simulink model "rocket"  (R2023a)
settings: Solver=FixedStepAuto  StartTime=0.0  StopTime=80  FixedStep=1/24  MaxStep=1.2  RelTol=1e-3
values from neighbouring files (symbols this model uses):
  arm_finne = 55    [rocket_variables.m]
  dry_mass = 25000    [rocket_variables.m]
  F_max = 845000    [rocket_variables.m]
  fuel_mass = 0    [rocket_variables.m]
  gravitational_constant = 6.6743E-11    (= 6.6743e-11)    [rocket_variables.m]
  h0 = 10000    [rocket_variables.m]
  h_ref = -1    [rocket_variables.m]
  J = dry_mass*L*L / 12    (= 10208333.3333)    [rocket_variables.m]
  k = 5.47    [rocket_variables.m]
  Kd1 = Kd    [rocket_variables.m]
  Kd_theta = 550000    [rocket_variables.m]
  Ki1 = Ki    [rocket_variables.m]
  Ki_theta = 125000    [rocket_variables.m]
  Kp1 = Kp    [rocket_variables.m]
  Kp_theta = 500000    [rocket_variables.m]
  mass_earth = 5.972E24    (= 5.972e+24)    [rocket_variables.m]
  mass_flow_engine = 1451.5    [rocket_variables.m]
  radius_earth = 6371000    [rocket_variables.m]
  theta_0 = pi/12    (= 0.261799387799)    [rocket_variables.m]
  theta_dot_0 = 0    [rocket_variables.m]
  theta_ref = 0    [rocket_variables.m]
  v_0 = -211    [rocket_variables.m]
libraries: embmathops x2
settings Model: Creator=eriknymobohne  LastModifiedBy=eriknymobohne

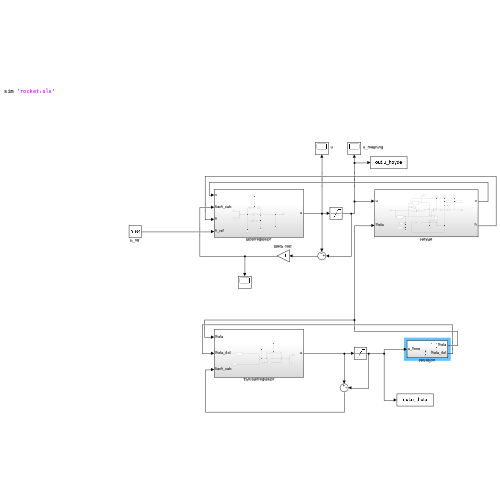
[thumbnail: Simulink's stored preview of the top-level diagram]
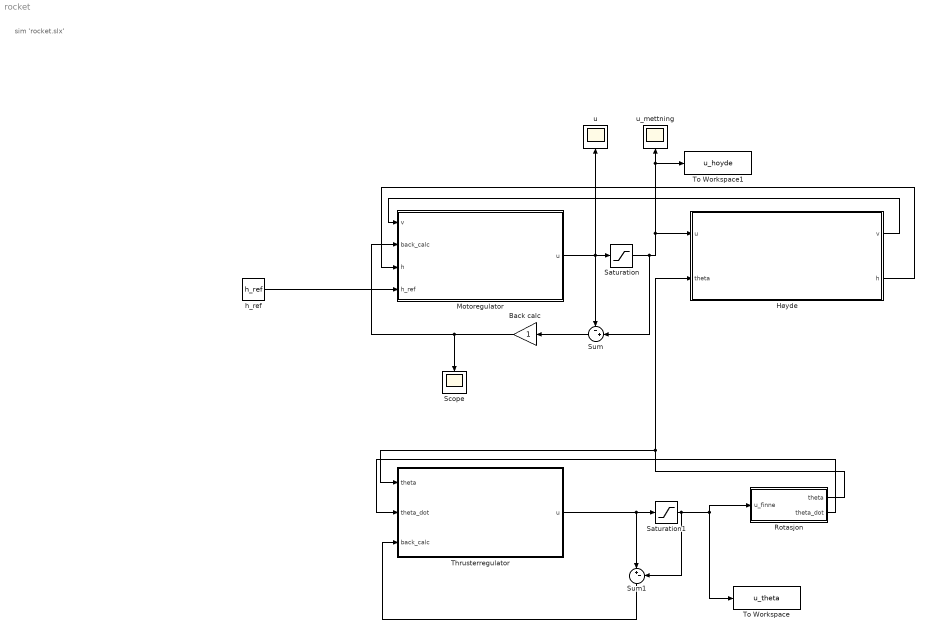
== system rocket ==
  note: sim 'rocket.slx'
  Back calc : Gain
  Høyde : Subsystem
  Motoregulator : Subsystem
  Rotasjon : Subsystem
  Saturation : Saturate  UpperLimit=F_max  LowerLimit=0
  Saturation1 : Saturate  UpperLimit=10000  LowerLimit=-10000
  Scope : Scope
  Sum : Sum  Inputs=-+|
  Sum1 : Sum  Inputs=|+-
  Thrusterregulator : Subsystem
  To Workspace : ToWorkspace  VariableName=u_theta  SaveFormat=Timeseries  SampleTime=-1
  To Workspace1 : ToWorkspace  VariableName=u_hoyde  SaveFormat=Timeseries  SampleTime=-1
  h_ref : Constant  Value=h_ref
  u : Scope
  u_mettning : Scope
  wires:
  Motoregulator/1(u) -> Saturation/1, Sum/1, u/1
  Saturation/1 -> To Workspace1/1, u_mettning/1, Høyde/1(u), Sum/2
  Sum/1 -> Back calc/1
  Back calc/1 -> Motoregulator/2(back_calc), Scope/1
  Høyde/2(h) -> Motoregulator/3(h)
  h_ref/1 -> Motoregulator/4(h_ref)
  Høyde/1(v) -> Motoregulator/1(v)
  Thrusterregulator/1(u) -> Sum1/1, Saturation1/1
  Sum1/1 -> Thrusterregulator/3(back_calc)
  Rotasjon/1(theta) -> Høyde/2(theta), Thrusterregulator/1(theta)
  Rotasjon/2(theta_dot) -> Thrusterregulator/2(theta_dot)
  Saturation1/1 -> Sum1/2, To Workspace/1, Rotasjon/1(u_finne)

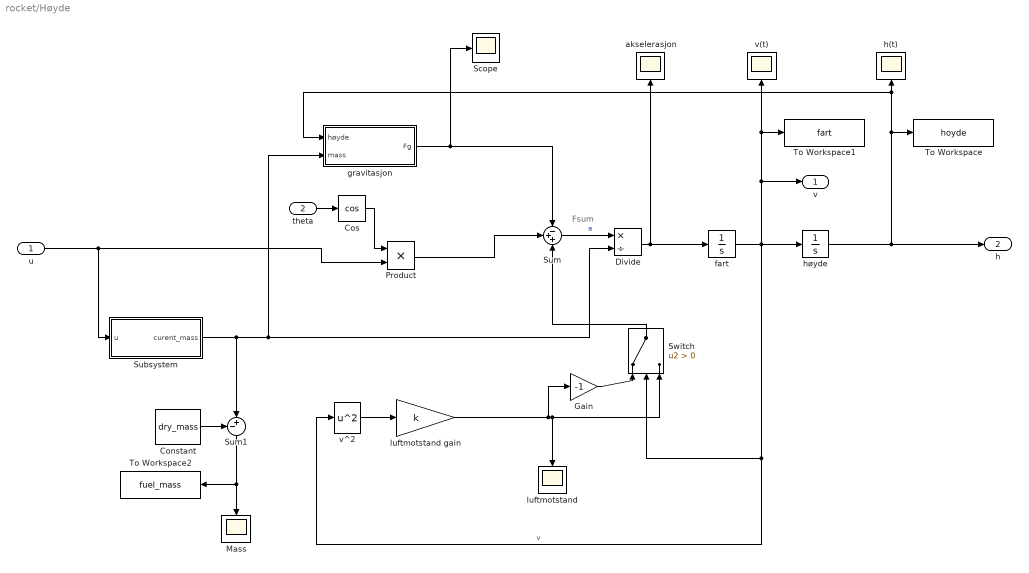
== system rocket/Høyde ==
  note: Fsum
  u : Inport
  theta : Inport  Port=2
  Constant : Constant  Value=dry_mass
  Cos : Trigonometry  Operator=cos
  Divide : Product  Inputs=*/
  Gain : Gain  Gain=-1
  Mass : Scope
  Product : Product
  Scope : Scope
  Subsystem : Subsystem
  Sum : Sum  Inputs=-++
  Sum1 : Sum  Inputs=-+|
  Switch : Switch  Criteria=u2 > Threshold  SaturateOnIntegerOverflow=off  InputSameDT=off
  To Workspace : ToWorkspace  VariableName=hoyde  SaveFormat=Timeseries  SampleTime=-1
  To Workspace1 : ToWorkspace  VariableName=fart  SaveFormat=Timeseries  SampleTime=-1
  To Workspace2 : ToWorkspace  VariableName=fuel_mass  SaveFormat=Timeseries  SampleTime=-1
  akselerasjon : Scope
  fart : Integrator  InitialCondition=v_0
  gravitasjon : Subsystem
  h(t) : Scope
  høyde : Integrator  InitialCondition=h0
  luftmotstand : Scope
  luftmotstand gain : Gain  Gain=k
  v(t) : Scope
  v^2 : Math  Operator=square
  v : Outport
  h : Outport  Port=2
  wires:
  fart/1 -> Switch/2, v^2/1, v/1, v(t)/1, To Workspace1/1, høyde/1  "v"
  v^2/1 -> luftmotstand gain/1
  luftmotstand gain/1 -> Switch/3, luftmotstand/1, Gain/1
  høyde/1 -> h/1, gravitasjon/1(høyde), h(t)/1, To Workspace/1
  Product/1 -> Sum/2
  theta/1 -> Cos/1
  u/1 -> Subsystem/1(u), Product/2
  Cos/1 -> Product/1
  gravitasjon/1(Fg) -> Scope/1, Sum/1
  Sum/1 -> Divide/1  "a"
  Subsystem/1(curent_mass) -> Sum1/2, Divide/2, gravitasjon/2(mass)
  Divide/1 -> fart/1, akselerasjon/1
  Switch/1 -> Sum/3
  Gain/1 -> Switch/1
  Constant/1 -> Sum1/1
  Sum1/1 -> To Workspace2/1, Mass/1

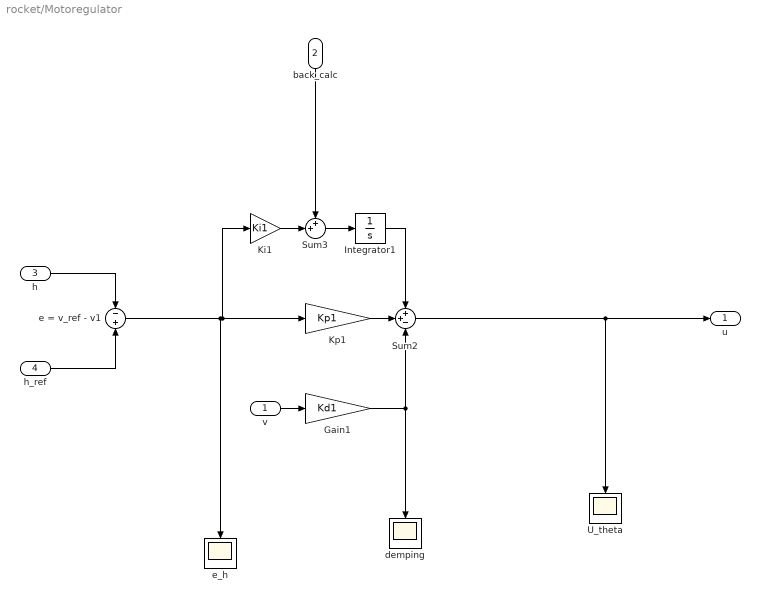
== system rocket/Motoregulator ==
  v : Inport
  back_calc : Inport  Port=2
  h : Inport  Port=3
  h_ref : Inport  Port=4
  Gain1 : Gain  Gain=Kd1
  Integrator1 : Integrator
  Ki1 : Gain  Gain=Ki1
  Kp1 : Gain  Gain=Kp1
  Sum2 : Sum  Inputs=++-
  Sum3 : Sum  Inputs=++|
  U_theta : Scope
  demping : Scope
  e = v_ref - v1 : Sum  Inputs=-|+
  e_h : Scope
  u : Outport
  wires:
  Integrator1/1 -> Sum2/1
  e = v_ref - v1/1 -> Ki1/1, Kp1/1, e_h/1
  Sum3/1 -> Integrator1/1
  h/1 -> e = v_ref - v1/1
  Kp1/1 -> Sum2/2
  Ki1/1 -> Sum3/2
  h_ref/1 -> e = v_ref - v1/2
  Sum2/1 -> U_theta/1, u/1
  back_calc/1 -> Sum3/1
  v/1 -> Gain1/1
  Gain1/1 -> Sum2/3, demping/1

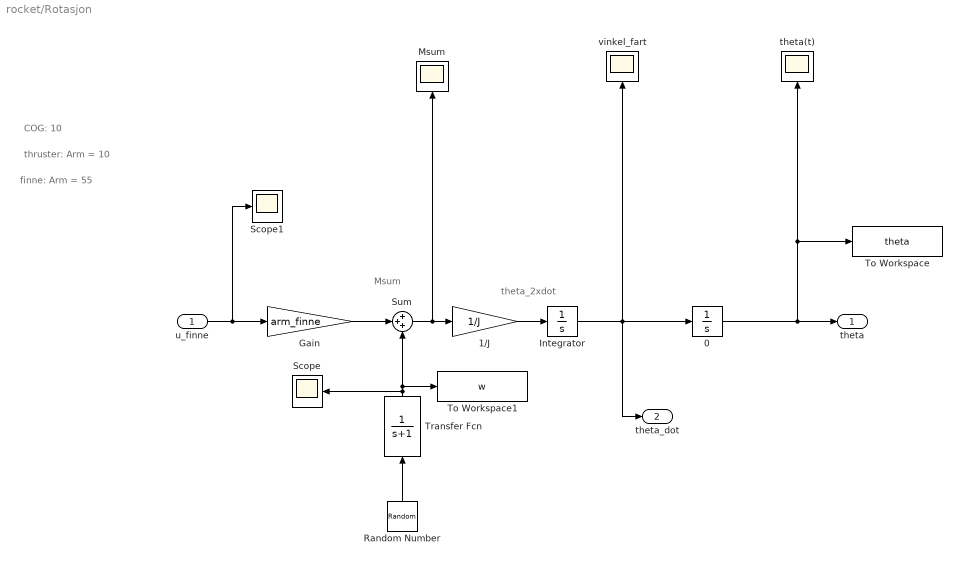
== system rocket/Rotasjon ==
  note: finne: Arm = 55
  note: COG: 10
  note: thruster: Arm = 10
  note: theta_2xdot
  note: Msum
  u_finne : Inport
  0 : Integrator  InitialCondition=theta_0
  1/J : Gain  Gain=1/J
  Gain : Gain  Gain=arm_finne
  Integrator : Integrator  InitialCondition=theta_dot_0
  Msum : Scope
  Random Number : RandomNumber  Mean=1000/2  Variance=10000000000  Seed=100000  SampleTime=1/24
  Scope : Scope
  Scope1 : Scope
  Sum : Sum  Inputs=+++
  To Workspace : ToWorkspace  VariableName=theta  SaveFormat=Timeseries  SampleTime=-1
  To Workspace1 : ToWorkspace  VariableName=w  SaveFormat=Timeseries  SampleTime=-1
  Transfer Fcn : TransferFcn  Denominator=[1 1]
  theta(t) : Scope
  vinkel_fart : Scope
  theta : Outport
  theta_dot : Outport  Port=2
  wires:
  0/1 -> theta(t)/1, To Workspace/1, theta/1
  Integrator/1 -> 0/1, vinkel_fart/1, theta_dot/1
  Sum/1 -> Msum/1, 1/J/1
  1/J/1 -> Integrator/1
  u_finne/1 -> Scope1/1, Gain/1
  Gain/1 -> Sum/2
  Random Number/1 -> Transfer Fcn/1
  Transfer Fcn/1 -> Sum/3, To Workspace1/1, Scope/1

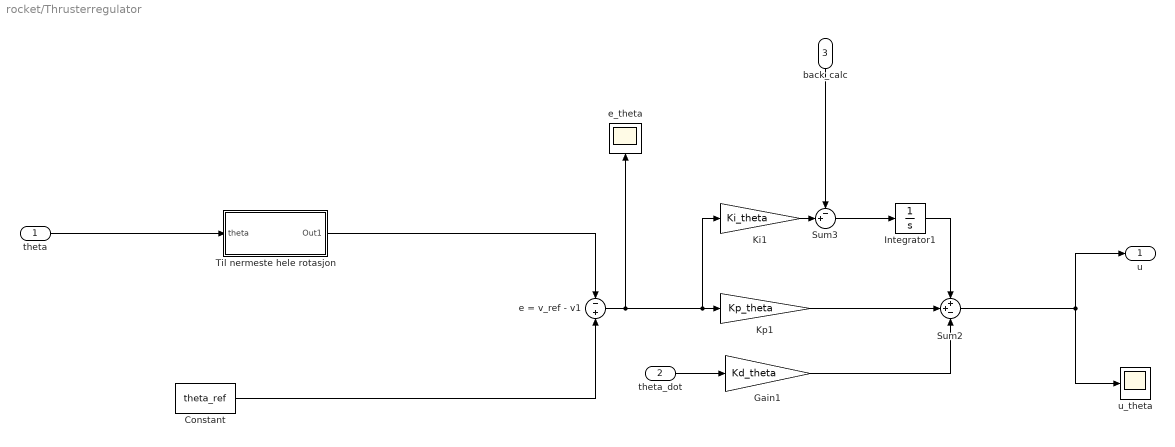
== system rocket/Thrusterregulator ==
  theta : Inport
  theta_dot : Inport  Port=2
  back_calc : Inport  Port=3
  Constant : Constant  Value=theta_ref
  Gain1 : Gain  Gain=Kd_theta
  Integrator1 : Integrator
  Ki1 : Gain  Gain=Ki_theta
  Kp1 : Gain  Gain=Kp_theta
  Sum2 : Sum  Inputs=++-
  Sum3 : Sum  Inputs=-+|
  Til nermeste hele rotasjon : Subsystem
  e = v_ref - v1 : Sum  Inputs=-|+
  e_theta : Scope
  u_theta : Scope
  u : Outport
  wires:
  Integrator1/1 -> Sum2/1
  e = v_ref - v1/1 -> Ki1/1, Kp1/1, e_theta/1
  Sum3/1 -> Integrator1/1
  Kp1/1 -> Sum2/2
  Ki1/1 -> Sum3/2
  Sum2/1 -> u/1, u_theta/1
  back_calc/1 -> Sum3/1
  theta_dot/1 -> Gain1/1
  Gain1/1 -> Sum2/3
  Constant/1 -> e = v_ref - v1/2
  theta/1 -> Til nermeste hele rotasjon/1(theta)
  Til nermeste hele rotasjon/1(Out1) -> e = v_ref - v1/1

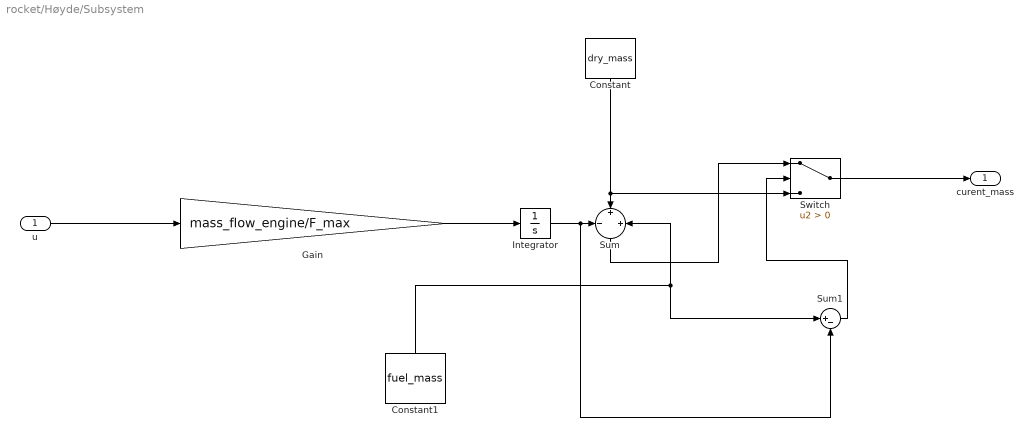
== system rocket/Høyde/Subsystem ==
  u : Inport
  Constant : Constant  Value=dry_mass
  Constant1 : Constant  Value=fuel_mass
  Gain : Gain  Gain=mass_flow_engine/F_max
  Integrator : Integrator
  Sum : Sum  Inputs=-|+|+
  Sum1 : Sum  Inputs=|+-
  Switch : Switch  Criteria=u2 > Threshold  SaturateOnIntegerOverflow=off  InputSameDT=off
  curent_mass : Outport
  wires:
  Gain/1 -> Integrator/1
  u/1 -> Gain/1
  Integrator/1 -> Sum1/2, Sum/1
  Constant/1 -> Switch/3, Sum/2
  Constant1/1 -> Sum1/1, Sum/3
  Sum1/1 -> Switch/2
  Switch/1 -> curent_mass/1
  Sum/1 -> Switch/1

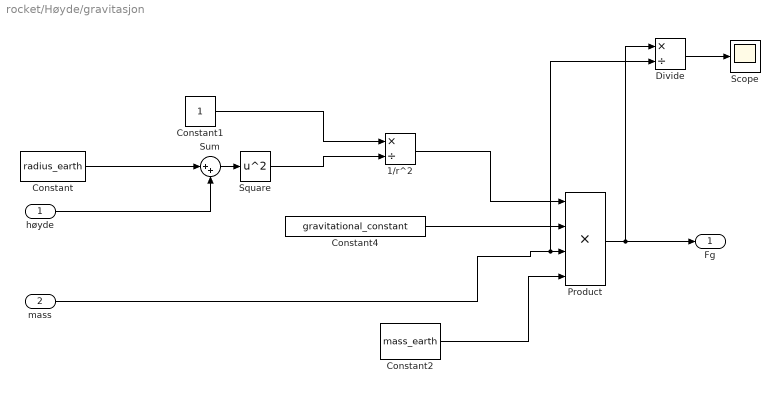
== system rocket/Høyde/gravitasjon ==
  høyde : Inport
  mass : Inport  Port=2
  1/r^2 : Product  Inputs=*/
  Constant : Constant  Value=radius_earth
  Constant1 : Constant
  Constant2 : Constant  Value=mass_earth
  Constant4 : Constant  Value=gravitational_constant
  Divide : Product  Inputs=*/
  Product : Product  Inputs=4
  Scope : Scope
  Square : Math  Operator=square
  Sum : Sum  Inputs=|++
  Fg : Outport
  wires:
  Constant/1 -> Sum/1
  høyde/1 -> Sum/2
  Sum/1 -> Square/1
  Square/1 -> 1/r^2/2
  Constant1/1 -> 1/r^2/1
  1/r^2/1 -> Product/1
  Constant4/1 -> Product/2
  Constant2/1 -> Product/4
  Product/1 -> Divide/1, Fg/1
  mass/1 -> Divide/2, Product/3
  Divide/1 -> Scope/1

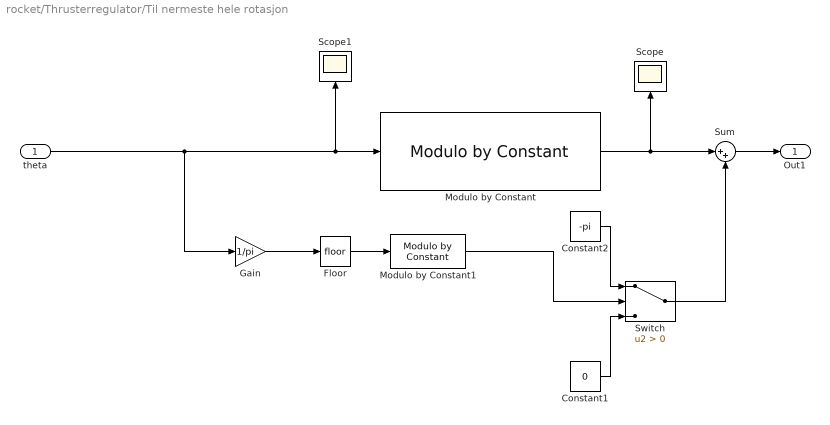
== system rocket/Thrusterregulator/Til nermeste hele rotasjon ==
  theta : Inport
  Constant1 : Constant  Value=0
  Constant2 : Constant  Value=-pi
  Floor : Rounding
  Gain : Gain  Gain=1/pi
  Modulo by Constant : embmathops/Modulo by Constant  Denominator=pi  SimulateUsing=Code generation
      settings: LibrarySourceBlock=embeddedMathLib/Modulo by Constant
  Modulo by Constant1 : embmathops/Modulo by Constant  Denominator=2  SimulateUsing=Code generation
      settings: LibrarySourceBlock=embeddedMathLib/Modulo by Constant
  Scope : Scope
  Scope1 : Scope
  Sum : Sum  Inputs=|++
  Switch : Switch  Criteria=u2 > Threshold  SaturateOnIntegerOverflow=off  InputSameDT=off
  Out1 : Outport
  wires:
  Constant1/1 -> Switch/3
  Constant2/1 -> Switch/1
  Modulo by Constant/1 -> Sum/1, Scope/1
  Switch/1 -> Sum/2
  theta/1 -> Modulo by Constant/1, Scope1/1, Gain/1
  Floor/1 -> Modulo by Constant1/1
  Gain/1 -> Floor/1
  Modulo by Constant1/1 -> Switch/2
  Sum/1 -> Out1/1
